simulink model "item2_simulink_motorCC_217947_222370"  (R2022a)
settings: Solver=VariableStepAuto  StartTime=0.0  StopTime=0.2  RelTol=1e-6
values from neighbouring files (symbols this model uses):
  B = 0    [matlab_motorCC_217947_222370.m]
  Ia_placa = 25    [matlab_motorCC_217947_222370.m]
  J = 0.00252    [matlab_motorCC_217947_222370.m]
  K = Te_placa/Ia_placa    (= 0.424752712124)    [matlab_motorCC_217947_222370.m]
  Kac = 1/Kpc    (= 0.588235294118)    [matlab_motorCC_217947_222370.m]
  Kas = 1/Kps    (= 1.68552663541)    [matlab_motorCC_217947_222370.m]
  Kic = Ra*wcc    (= 260)    [matlab_motorCC_217947_222370.m]
  Kis = J*wcs^2/(5*K)    (= 11.8657276485)    [matlab_motorCC_217947_222370.m]
  Kpc = La*wcc    (= 1.7)    [matlab_motorCC_217947_222370.m]
  Kps = J*wcs/K    (= 0.593286382423)    [matlab_motorCC_217947_222370.m]
  La = 1.7e-3    (= 0.0017)    [matlab_motorCC_217947_222370.m]
  Ra = 0.26    [matlab_motorCC_217947_222370.m]
  Te_placa = Potencia/Wm_placa    (= 10.6188178031)    [matlab_motorCC_217947_222370.m]
  Va_placa = 140    [matlab_motorCC_217947_222370.m]
libraries: spsTriangleGeneratorLib x1
settings Model: Creator=Pichau  LastModifiedBy=Pichau

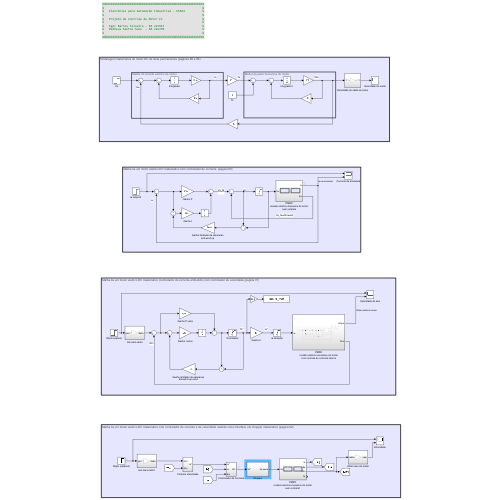
[thumbnail: Simulink's stored preview of the top-level diagram]
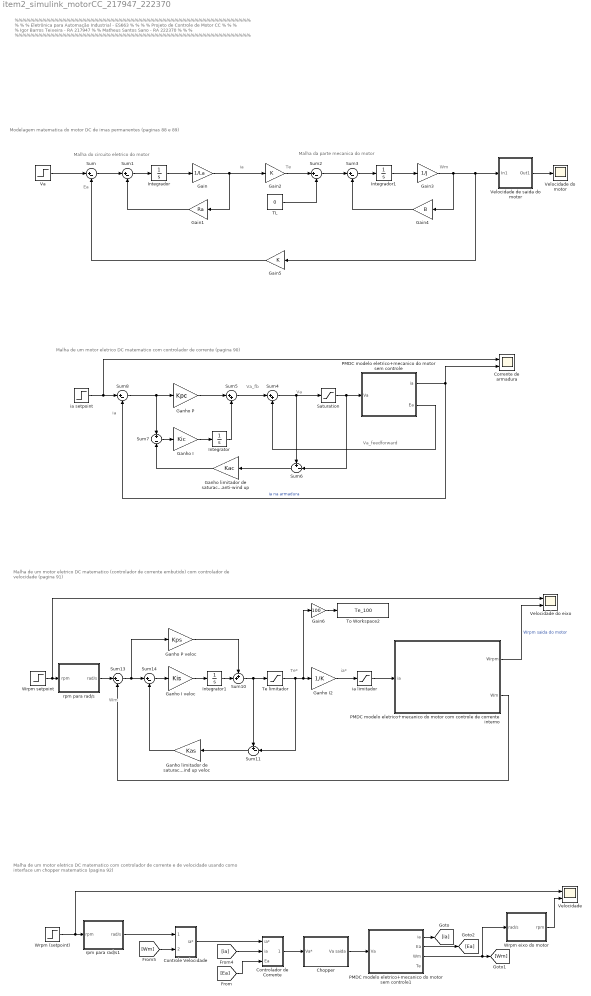
== system item2_simulink_motorCC_217947_222370 ==
  note: Malha de um motor eletrico DC matematico com controlador de corrente e de velocidade usando como interface um chopper matematico (pagina 92)
  note: Malha de um motor eletrico DC matematico (controlador de corrente embutido) com controlador de velocidade (pagina 91)
  note: Malha de um motor eletrico DC matematico com controlador de corrente (pagina 90)
  note: Modelagem matematica do motor DC de imas permanentes (paginas 88 e 89)
  note: Va
  note: Va_feedforward
  note: Malha da parte mecanica do motor
  note: Ea
  note: %%%%%%%%%%%%%%%%%%%%%%%%%%%%%%%%%%%%%%%%%%%%%%%%%%%%%%%%%%%
      | % %
      | % Eletrônica para Automação Industrial - ES663 %
      | % %
      | % Projeto de Controle de Motor CC %
      | % %
      | % Igor Barros Teixeira - RA 217947 %
      | % Matheus Santos Sano - RA 222370 %
      | % %
      | %%%%%%%%%%%%%%%%%%%%%%%%%%%%%%%%%%%%%%%%%%%%%%%%%%%%%%%%%%%
  note: Te
  note: Wm
  note: Malha do circuito eletrico do motor
  note: ia
  note: Va_fb
  note: ia
  note: Wm
  note: Te*
  note: ia*
  Chopper : Subsystem
  Controlador de Corrente : Subsystem
  Controle Velocidade : Subsystem
  Corrente de armadura : Scope  NumInputPorts=2
  Gain : Gain  Gain=1/La
  Gain1 : Gain  Gain=Ra
  Gain2 : Gain  Gain=K
  Gain3 : Gain  Gain=1/J
  Gain4 : Gain  Gain=B
  Gain5 : Gain  Gain=K
  Gain6 : Gain  Gain=100
  Ganho I : Gain  Gain=Kic
  Ganho I veloc : Gain  Gain=Kis
  Ganho I2 : Gain  Gain=1/K
  Ganho P : Gain  Gain=Kpc
  Ganho P veloc : Gain  Gain=Kps
  Ganho limitador de saturacao anti-wind up : Gain  Gain=Kac
  Ganho limitador de saturacao anti-wind up veloc : Gain  Gain=Kas
  Integrador : Integrator
  Integrador1 : Integrator
  Integrator : Integrator
  Integrator1 : Integrator
  PMDC modelo eletrico+mecanico do motor com controle de corrente interno : Subsystem
  PMDC modelo eletrico+mecanico do motor sem controle : Subsystem
  PMDC modelo eletrico+mecanico do motor sem controle1 : Subsystem
  Saturation : Saturate  UpperLimit=Va_placa  LowerLimit=-Va_placa
  Sum{,1..3,8,13..14} (7 alike) : Sum  Inputs=|+-
  Sum10 : Sum  Inputs=++|
  Sum11 : Sum  Inputs=+-|
  Sum4 : Sum  Inputs=|++
  Sum5 : Sum  Inputs=|++
  Sum6 : Sum  Inputs=+-|
  Sum7 : Sum  Inputs=+|-
  TL : Constant  Value=0
  Te limitador : Saturate  UpperLimit=Te_placa  LowerLimit=-Te_placa
  To Workspace2 : ToWorkspace  VariableName=Te_100  SaveFormat=Timeseries  SampleTime=-1
  Va : Step  Time=0.05  After=140  SampleTime=0
  Velocidade : Scope  NumInputPorts=2
  Velocidade de saida do motor : Subsystem
  Velocidade do eixo : Scope  NumInputPorts=2
  Velocidade do motor : Scope
  Wrpm (setpoint) : Step  Time=0.05  After=2500  SampleTime=0
  Wrpm eixo do motor : Subsystem
  Wrpm setpoint : Step  Time=0.05  After=2500  SampleTime=0
  ia limitador : Saturate  UpperLimit=Ia_placa  LowerLimit=-Ia_placa
  ia setpoint : Step  Time=0.005  After=20  SampleTime=0
  rpm para rad/s : Subsystem
  rpm para rad/s1 : Subsystem
  wires:
  Sum/1 -> Sum1/1
  Sum1/1 -> Integrador/1
  Integrador/1 -> Gain/1
  Gain1/1 -> Sum1/2
  Va/1 -> Sum/1
  Gain/1 -> Gain1/1, Gain2/1
  Sum3/1 -> Integrador1/1
  Sum2/1 -> Sum3/1
  Gain2/1 -> Sum2/1
  Gain3/1 -> Gain4/1, Velocidade de saida do motor/1(In1), Gain5/1
  Integrador1/1 -> Gain3/1
  Gain4/1 -> Sum3/2
  TL/1 -> Sum2/2
  Gain5/1 -> Sum/2
  Velocidade de saida do motor/1(Out1) -> Velocidade do motor/1
  Saturation/1 -> Sum6/2, PMDC modelo eletrico+mecanico do motor sem controle/1(Va)
  Sum4/1 -> Sum6/1, Saturation/1
  PMDC modelo eletrico+mecanico do motor sem controle/2(Ea) -> Sum4/2
  Sum5/1 -> Sum4/1
  Sum6/1 -> Ganho limitador de saturacao anti-wind up/1
  Sum7/1 -> Ganho I/1
  Ganho I/1 -> Integrator/1
  Integrator/1 -> Sum5/2
  Ganho limitador de saturacao anti-wind up/1 -> Sum7/2
  Ganho P/1 -> Sum5/1
  Sum8/1 -> Sum7/1, Ganho P/1
  PMDC modelo eletrico+mecanico do motor sem controle/1(ia) -> Sum8/2, Corrente de armadura/2  "ia na armadura"
  ia setpoint/1 -> Corrente de armadura/1, Sum8/1
  PMDC modelo eletrico+mecanico do motor com controle de corrente interno/2(Wm) -> Sum13/2
  Sum10/1 -> Sum11/1, Te limitador/1
  Ganho I veloc/1 -> Integrator1/1
  Te limitador/1 -> Gain6/1, Ganho I2/1, Sum11/2
  Sum11/1 -> Ganho limitador de saturacao anti-wind up veloc/1
  Wrpm setpoint/1 -> Velocidade do eixo/1, rpm para rad/s/1(rpm)
  rpm para rad/s/1(rad/s) -> Sum13/1
  Sum13/1 -> Ganho P veloc/1, Sum14/1
  Sum14/1 -> Ganho I veloc/1
  Ganho I2/1 -> ia limitador/1
  ia limitador/1 -> PMDC modelo eletrico+mecanico do motor com controle de corrente interno/1(ia)
  Integrator1/1 -> Sum10/2
  Ganho P veloc/1 -> Sum10/1
  Ganho limitador de saturacao anti-wind up veloc/1 -> Sum14/2
  Gain6/1 -> To Workspace2/1
  [ia] -> Controlador de Corrente/2(ia)
  [Wm] -> Controle Velocidade/2(Wm)
  rpm para rad/s1/1(rad/s) -> Controle Velocidade/1(Wm*)
  Wrpm (setpoint)/1 -> Velocidade/1, rpm para rad/s1/1(rpm)
  Controle Velocidade/1(ia*) -> Controlador de Corrente/1(ia*)
  PMDC modelo eletrico+mecanico do motor sem controle1/1(ia) -> [ia]
  PMDC modelo eletrico+mecanico do motor sem controle1/3(Wm) -> Wrpm eixo do motor/1(rad/s), [Wm]
  PMDC modelo eletrico+mecanico do motor sem controle1/2(Ea) -> [Ea]
  [Ea] -> Controlador de Corrente/3(Ea)
  Chopper/1(Va saida) -> PMDC modelo eletrico+mecanico do motor sem controle1/1(Va)
  Controlador de Corrente/1(Va*) -> Chopper/1(Va*)
  Wrpm eixo do motor/1(rpm) -> Velocidade/2
  PMDC modelo eletrico+mecanico do motor com controle de corrente interno/1(Wrpm) -> Velocidade do eixo/2  "Wrpm saida do motor"

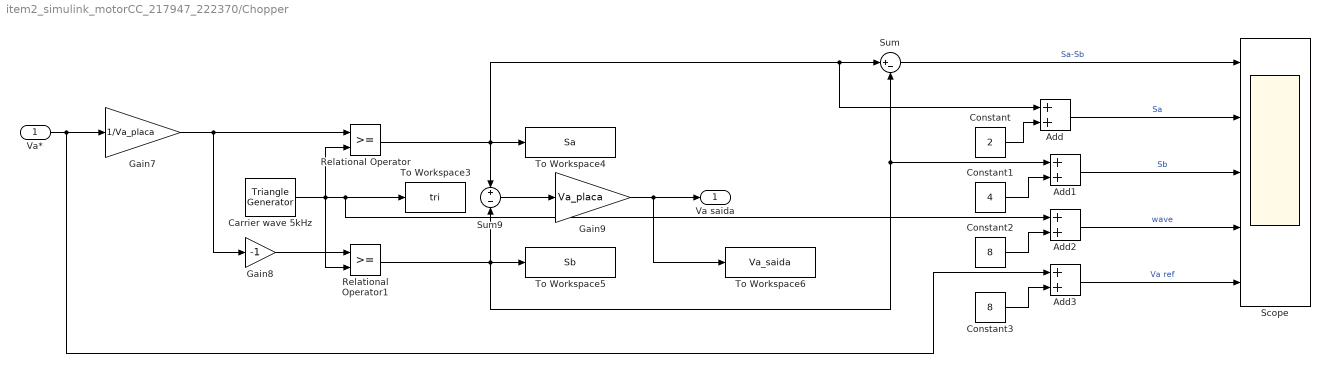
== system item2_simulink_motorCC_217947_222370/Chopper ==
  Va* : Inport
  Add{,1..3} (4 alike) : Sum
  Carrier wave 5kHz : spsTriangleGeneratorLib/Triangle Generator  Freq=5e3  Phase=0  Ts=0
  Constant : Constant  Value=2
  Constant1 : Constant  Value=4
  Constant2 : Constant  Value=8
  Constant3 : Constant  Value=8
  Gain7 : Gain  Gain=1/Va_placa
  Gain8 : Gain  Gain=-1
  Gain9 : Gain  Gain=Va_placa
  Relational Operator : RelationalOperator  OutDataTypeStr=boolean  RndMeth=Simplest  InputSameDT=off
  Relational Operator1 : RelationalOperator  OutDataTypeStr=boolean  RndMeth=Simplest  InputSameDT=off
  Scope : Scope  NumInputPorts=5
  Sum : Sum  Inputs=|+-
  Sum9 : Sum  Inputs=+|-
  To Workspace3 : ToWorkspace  VariableName=tri  SaveFormat=Timeseries  SampleTime=-1
  To Workspace4 : ToWorkspace  VariableName=Sa  SaveFormat=Timeseries  SampleTime=-1
  To Workspace5 : ToWorkspace  VariableName=Sb  SaveFormat=Timeseries  SampleTime=-1
  To Workspace6 : ToWorkspace  VariableName=Va_saida  SaveFormat=Timeseries  SampleTime=-1
  Va saida : Outport
  wires:
  Gain8/1 -> Relational Operator1/1
  Relational Operator/1 -> Add/1, Sum/1, Sum9/1, To Workspace4/1
  Gain9/1 -> Va saida/1, To Workspace6/1
  Carrier wave 5kHz/1 -> Add2/1, To Workspace3/1, Relational Operator/2, Relational Operator1/2
  Va*/1 -> Add3/1, Gain7/1
  Relational Operator1/1 -> Sum9/2, Sum/2, Add1/1, To Workspace5/1
  Sum9/1 -> Gain9/1
  Gain7/1 -> Gain8/1, Relational Operator/1
  Sum/1 -> Scope/1  "Sa-Sb"
  Add/1 -> Scope/2  "Sa"
  Constant/1 -> Add/2
  Constant1/1 -> Add1/2
  Add1/1 -> Scope/3  "Sb"
  Constant2/1 -> Add2/2
  Add2/1 -> Scope/4  "wave"
  Constant3/1 -> Add3/2
  Add3/1 -> Scope/5  "Va ref"

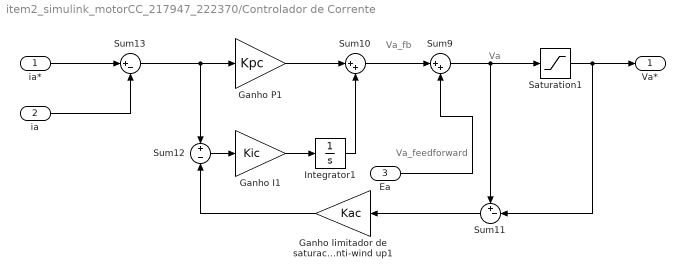
== system item2_simulink_motorCC_217947_222370/Controlador de Corrente ==
  note: Va
  note: Va_feedforward
  note: Va_fb
  ia* : Inport
  ia : Inport  Port=2
  Ea : Inport  Port=3
  Ganho I1 : Gain  Gain=Kic
  Ganho P1 : Gain  Gain=Kpc
  Ganho limitador de saturacao anti-wind up1 : Gain  Gain=Kac
  Integrator1 : Integrator
  Saturation1 : Saturate  UpperLimit=Va_placa  LowerLimit=-Va_placa
  Sum10 : Sum  Inputs=|++
  Sum11 : Sum  Inputs=+-|
  Sum12 : Sum  Inputs=+|-
  Sum13 : Sum  Inputs=|+-
  Sum9 : Sum  Inputs=|++
  Va* : Outport
  wires:
  Sum9/1 -> Sum11/1, Saturation1/1
  Sum10/1 -> Sum9/1
  Sum13/1 -> Sum12/1, Ganho P1/1
  Ganho P1/1 -> Sum10/1
  Sum12/1 -> Ganho I1/1
  Sum11/1 -> Ganho limitador de saturacao anti-wind up1/1
  Ganho I1/1 -> Integrator1/1
  ia*/1 -> Sum13/1
  Integrator1/1 -> Sum10/2
  Ganho limitador de saturacao anti-wind up1/1 -> Sum12/2
  Saturation1/1 -> Va*/1, Sum11/2
  ia/1 -> Sum13/2
  Ea/1 -> Sum9/2

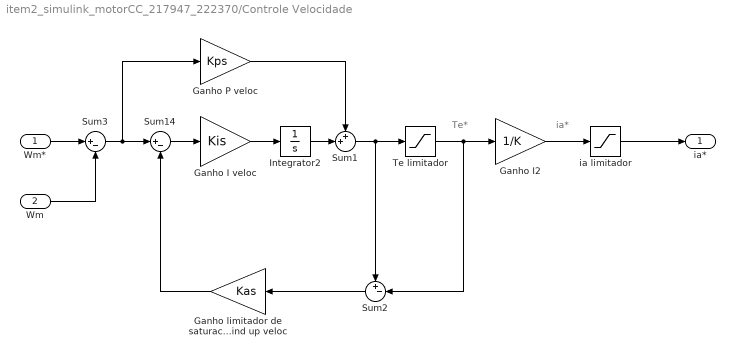
== system item2_simulink_motorCC_217947_222370/Controle Velocidade ==
  note: Te*
  note: ia*
  Wm* : Inport
  Wm : Inport  Port=2
  Ganho I veloc : Gain  Gain=Kis
  Ganho I2 : Gain  Gain=1/K
  Ganho P veloc : Gain  Gain=Kps
  Ganho limitador de saturacao anti-wind up veloc : Gain  Gain=Kas
  Integrator2 : Integrator
  Sum1 : Sum  Inputs=++|
  Sum14 : Sum  Inputs=|+-
  Sum2 : Sum  Inputs=+-|
  Sum3 : Sum  Inputs=|+-
  Te limitador : Saturate  UpperLimit=Te_placa  LowerLimit=-Te_placa
  ia limitador : Saturate  UpperLimit=Ia_placa  LowerLimit=-Ia_placa
  ia* : Outport
  wires:
  Ganho I2/1 -> ia limitador/1
  Sum3/1 -> Ganho P veloc/1, Sum14/1
  Sum14/1 -> Ganho I veloc/1
  Te limitador/1 -> Ganho I2/1, Sum2/2
  Ganho limitador de saturacao anti-wind up veloc/1 -> Sum14/2
  Ganho P veloc/1 -> Sum1/1
  Sum1/1 -> Sum2/1, Te limitador/1
  Integrator2/1 -> Sum1/2
  Wm*/1 -> Sum3/1
  Sum2/1 -> Ganho limitador de saturacao anti-wind up veloc/1
  Ganho I veloc/1 -> Integrator2/1
  ia limitador/1 -> ia*/1
  Wm/1 -> Sum3/2

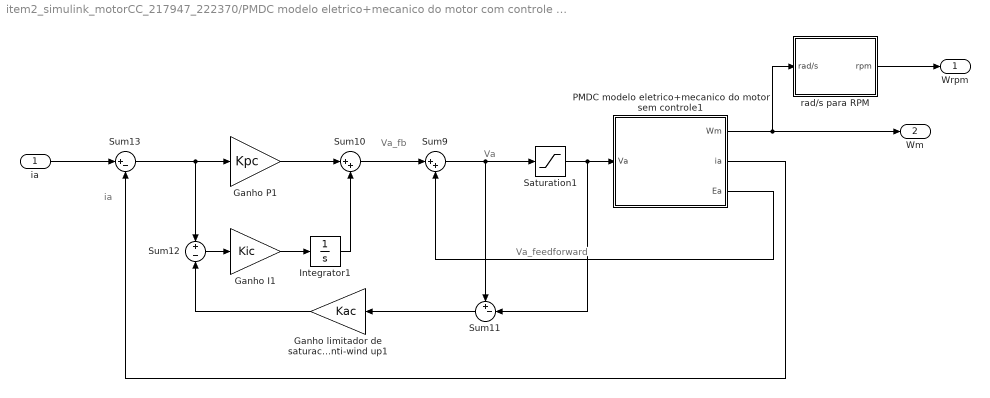
== system item2_simulink_motorCC_217947_222370/PMDC modelo eletrico+mecanico do motor com controle de corrente interno ==
  note: Va_feedforward
  note: Va
  note: ia
  note: Va_fb
  ia : Inport
  Ganho I1 : Gain  Gain=Kic
  Ganho P1 : Gain  Gain=Kpc
  Ganho limitador de saturacao anti-wind up1 : Gain  Gain=Kac
  Integrator1 : Integrator
  PMDC modelo eletrico+mecanico do motor sem controle1 : Subsystem
  Saturation1 : Saturate  UpperLimit=Va_placa  LowerLimit=-Va_placa
  Sum10 : Sum  Inputs=|++
  Sum11 : Sum  Inputs=+-|
  Sum12 : Sum  Inputs=+|-
  Sum13 : Sum  Inputs=|+-
  Sum9 : Sum  Inputs=|++
  rad/s para RPM : Subsystem
  Wrpm : Outport
  Wm : Outport  Port=2
  wires:
  PMDC modelo eletrico+mecanico do motor sem controle1/3(Ea) -> Sum9/2
  Sum10/1 -> Sum9/1
  Ganho limitador de saturacao anti-wind up1/1 -> Sum12/2
  Sum9/1 -> Sum11/1, Saturation1/1
  Sum12/1 -> Ganho I1/1
  Sum11/1 -> Ganho limitador de saturacao anti-wind up1/1
  Integrator1/1 -> Sum10/2
  Saturation1/1 -> Sum11/2, PMDC modelo eletrico+mecanico do motor sem controle1/1(Va)
  Ganho P1/1 -> Sum10/1
  Ganho I1/1 -> Integrator1/1
  PMDC modelo eletrico+mecanico do motor sem controle1/2(ia) -> Sum13/2
  Sum13/1 -> Sum12/1, Ganho P1/1
  ia/1 -> Sum13/1
  PMDC modelo eletrico+mecanico do motor sem controle1/1(Wm) -> rad/s para RPM/1(rad/s), Wm/1
  rad/s para RPM/1(rpm) -> Wrpm/1

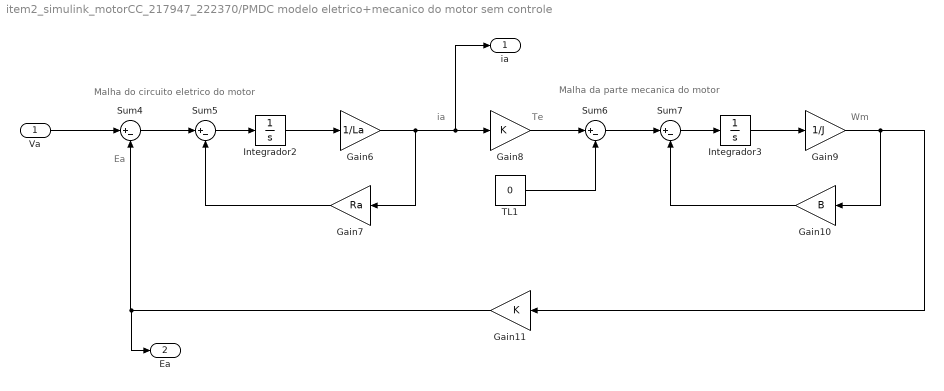
== system item2_simulink_motorCC_217947_222370/PMDC modelo eletrico+mecanico do motor sem controle ==
  note: Malha da parte mecanica do motor
  note: Malha do circuito eletrico do motor
  note: ia
  note: Te
  note: Wm
  note: Ea
  Va : Inport
  Gain10 : Gain  Gain=B
  Gain11 : Gain  Gain=K
  Gain6 : Gain  Gain=1/La
  Gain7 : Gain  Gain=Ra
  Gain8 : Gain  Gain=K
  Gain9 : Gain  Gain=1/J
  Integrador2 : Integrator
  Integrador3 : Integrator
  Sum{4..7} (4 alike) : Sum  Inputs=|+-
  TL1 : Constant  Value=0
  ia : Outport
  Ea : Outport  Port=2
  wires:
  Sum6/1 -> Sum7/1
  Gain6/1 -> Gain7/1, ia/1, Gain8/1
  Gain9/1 -> Gain10/1, Gain11/1
  Gain10/1 -> Sum7/2
  Sum7/1 -> Integrador3/1
  Sum4/1 -> Sum5/1
  TL1/1 -> Sum6/2
  Integrador3/1 -> Gain9/1
  Sum5/1 -> Integrador2/1
  Gain11/1 -> Ea/1, Sum4/2
  Gain8/1 -> Sum6/1
  Integrador2/1 -> Gain6/1
  Gain7/1 -> Sum5/2
  Va/1 -> Sum4/1

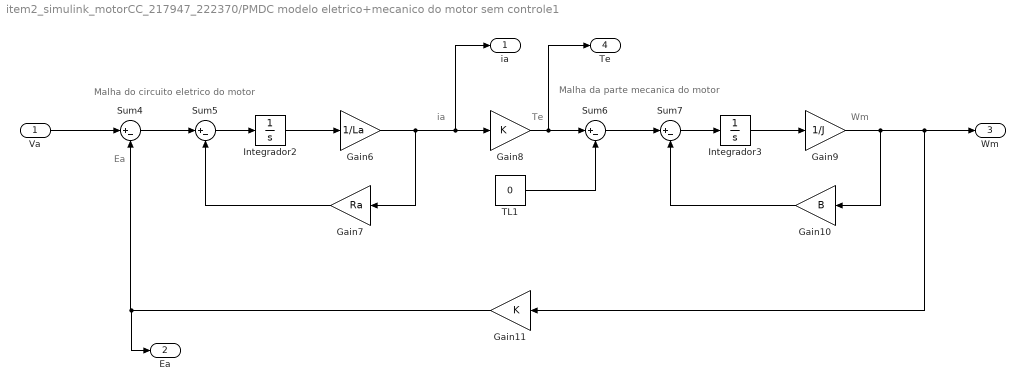
== system item2_simulink_motorCC_217947_222370/PMDC modelo eletrico+mecanico do motor sem controle1 ==
  note: Malha da parte mecanica do motor
  note: Malha do circuito eletrico do motor
  note: ia
  note: Te
  note: Wm
  note: Ea
  Va : Inport
  Gain10 : Gain  Gain=B
  Gain11 : Gain  Gain=K
  Gain6 : Gain  Gain=1/La
  Gain7 : Gain  Gain=Ra
  Gain8 : Gain  Gain=K
  Gain9 : Gain  Gain=1/J
  Integrador2 : Integrator
  Integrador3 : Integrator
  Sum{4..7} (4 alike) : Sum  Inputs=|+-
  TL1 : Constant  Value=0
  ia : Outport
  Ea : Outport  Port=2
  Wm : Outport  Port=3
  Te : Outport  Port=4
  wires:
  Sum6/1 -> Sum7/1
  Gain6/1 -> Gain7/1, ia/1, Gain8/1
  Gain9/1 -> Gain10/1, Wm/1, Gain11/1
  Gain10/1 -> Sum7/2
  Sum7/1 -> Integrador3/1
  Sum4/1 -> Sum5/1
  TL1/1 -> Sum6/2
  Integrador3/1 -> Gain9/1
  Sum5/1 -> Integrador2/1
  Gain11/1 -> Ea/1, Sum4/2
  Gain8/1 -> Te/1, Sum6/1
  Integrador2/1 -> Gain6/1
  Gain7/1 -> Sum5/2
  Va/1 -> Sum4/1

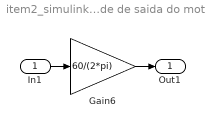
== system item2_simulink_motorCC_217947_222370/Velocidade de saida do motor ==
  In1 : Inport
  Gain6 : Gain  Gain=60/(2*pi)
  Out1 : Outport
  wires:
  In1/1 -> Gain6/1
  Gain6/1 -> Out1/1

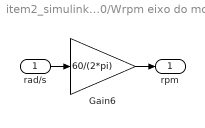
== system item2_simulink_motorCC_217947_222370/Wrpm eixo do motor ==
  rad/s : Inport
  Gain6 : Gain  Gain=60/(2*pi)
  rpm : Outport
  wires:
  rad/s/1 -> Gain6/1
  Gain6/1 -> rpm/1

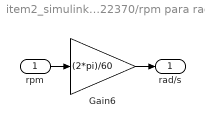
== system item2_simulink_motorCC_217947_222370/rpm para rad//s ==
  rpm : Inport
  Gain6 : Gain  Gain=(2*pi)/60
  rad/s : Outport
  wires:
  rpm/1 -> Gain6/1
  Gain6/1 -> rad/s/1

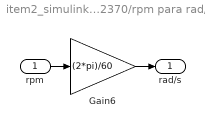
== system item2_simulink_motorCC_217947_222370/rpm para rad//s1 ==
  rpm : Inport
  Gain6 : Gain  Gain=(2*pi)/60
  rad/s : Outport
  wires:
  rpm/1 -> Gain6/1
  Gain6/1 -> rad/s/1

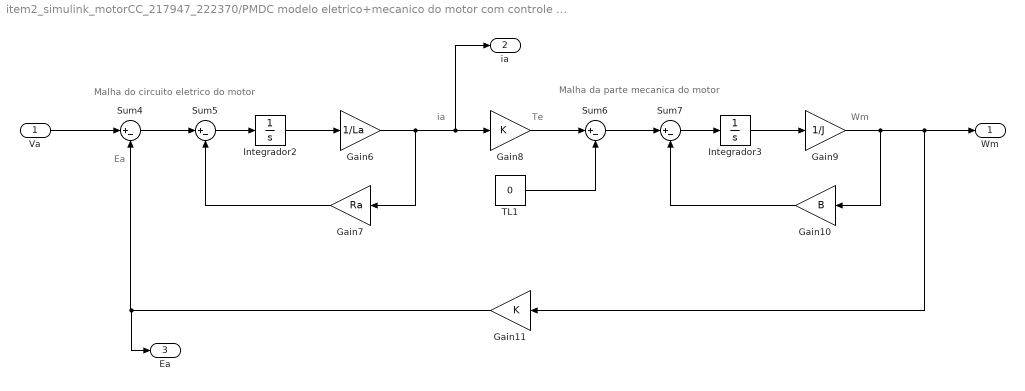
== system item2_simulink_motorCC_217947_222370/PMDC modelo eletrico+mecanico do motor com controle de corrente interno/PMDC modelo eletrico+mecanico do motor sem controle1 ==
  note: Malha da parte mecanica do motor
  note: Malha do circuito eletrico do motor
  note: ia
  note: Te
  note: Wm
  note: Ea
  Va : Inport
  Gain10 : Gain  Gain=B
  Gain11 : Gain  Gain=K
  Gain6 : Gain  Gain=1/La
  Gain7 : Gain  Gain=Ra
  Gain8 : Gain  Gain=K
  Gain9 : Gain  Gain=1/J
  Integrador2 : Integrator
  Integrador3 : Integrator
  Sum{4..7} (4 alike) : Sum  Inputs=|+-
  TL1 : Constant  Value=0
  Wm : Outport
  ia : Outport  Port=2
  Ea : Outport  Port=3
  wires:
  Sum6/1 -> Sum7/1
  Gain6/1 -> Gain7/1, ia/1, Gain8/1
  Gain9/1 -> Gain10/1, Wm/1, Gain11/1
  Gain10/1 -> Sum7/2
  Sum7/1 -> Integrador3/1
  Sum4/1 -> Sum5/1
  TL1/1 -> Sum6/2
  Integrador3/1 -> Gain9/1
  Sum5/1 -> Integrador2/1
  Gain11/1 -> Ea/1, Sum4/2
  Gain8/1 -> Sum6/1
  Integrador2/1 -> Gain6/1
  Gain7/1 -> Sum5/2
  Va/1 -> Sum4/1

== system item2_simulink_motorCC_217947_222370/PMDC modelo eletrico+mecanico do motor com controle de corrente interno/rad//s para RPM ==
  rad/s : Inport
  Gain6 : Gain  Gain=60/(2*pi)
  rpm : Outport
  wires:
  rad/s/1 -> Gain6/1
  Gain6/1 -> rpm/1
